simulink library "DAQ_lib_HallPositionTorque"  (R2014b)
settings: Solver=ode45  StartTime=0.0  StopTime=10.0  RelTol=1e-3
undefined symbols (not defined in the file): A_lpf_velocity, ANOMALY_INIT, B1_lpf_velocity, B2_lpf_velocity, Calibration, EnableFT, EncoderAngleLimits, EncoderFiltSys, EncoderThreshold, FTCalibration, GearOffsets, IMUAngleLimits, IMUCommand, IMUThreshold, IMUTorsoOffsets, m_XR17D15x, MAX_ANOMALY, MedullaCommand, MicrostrainFiltSys, MODBUS_TIMEOUT, ResetDAQ, ResetYaw, sample_time, standard, STREAMING_TIMEOUT, TareFT, TorsoCOMOffsets, Ts, TsCAN, TsKVH, UseMicrostrainRate
libraries: xpcethercatlib x207, simulink x53, canmsglib x21, speedgoatlib x13, slrtlib x5, speedgoatlib_IO601 x5, dspswit3 x2, dspmtrx3 x2, xpcseriallib x1, SpeedgoatModified x1
(part 2 of 7)

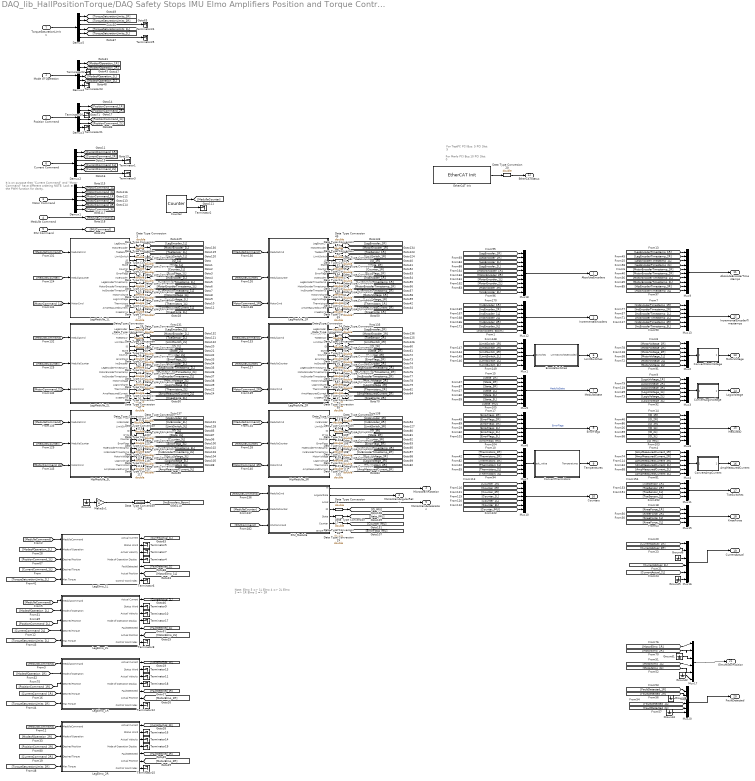
== system DAQ_lib_HallPositionTorque/DAQ Safety Stops IMU Elmo Amplifiers Position and Torque Control with Hall Sensors/DAQ/EtherCATNetwork/EtherCATRobotMicrostrain ==
  note: It is on purpose that "Current Command"
      | and "Motor Command" have different ordering
      | NOTE: Look at the PWM function for clarity.
  note: Note:
      | Elmo 5 => 1L
      | Elmo 4 => 2L
      | Elmo 3 => 1R
      | Elmo 2 => 2R
  note: For Marlo
      | PCI Bus:10 PCI Slot: 0
  note: For TestPC
      | PCI Bus: 5 PCI Slot: 5
  Mode of Operation : Inport
  Position Command : Inport  Port=2
  Motor Command : Inport  Port=3
  Medulla Command : Inport  Port=4
  IMU Command : Inport  Port=5
  Current Command : Inport  Port=6
  TorqueSaturationLimits : Inport  Port=7
  ConvertAmpCurrent : MATLAB Function  TreatAsAtomicUnit=on
  ConvertLogicVoltage : MATLAB Function  TreatAsAtomicUnit=on
  ConvertMotorVoltage : MATLAB Function  TreatAsAtomicUnit=on
  ConvertThermistors : MATLAB Function  TreatAsAtomicUnit=on
  Counter : dspswit3/Counter  Direction=Up  CountEvent=Free running  CounterSize=User defined  MaxCount=65535  InitialCount=0  Output=Count and Hit  HitValue=32  ResetInput=off  SamplesPerFrame=1  Ts=Ts  CntDtype=double  HitDtype=Logical
  Data Type Conversion{1..21,23,25..39,45,47,49..63,69,71,73..87,93,95,98,101..112,114,116..126,141,157} (100 alike) : DataTypeConversion  OutDataTypeStr=double
  Demux{1..5} (5 alike) : Demux  Outputs=6
  EncodeSwitches : MATLAB Function  TreatAsAtomicUnit=on
  "EtherCAT Init " : xpcethercatlib/EtherCAT Init   Priority=0  config_file=C:\Users\rosshart\Desktop\ATRIAS_SVN\MARLO_3D_Controllers\DAQ_withElmos\500us\AllMedullasWithAllMotors_07_08_2015_withBoom.eni.xml  device_id=0  pci_bus=10  pci_slot=0  enaDebug=off  enaDC=on  errLink=off  masterDbg=off  stateChgDbg=off  baseClock=off  masterCfg=off  logFile='c:\dbglog.txt'  sample_time=0.000500
  Ground{,1..6} (7 alike) : Ground
  HipMedulla_3L : Subsystem
  HipMedulla_3R : Subsystem
  IMU_Medulla : Subsystem
  LegElmo_1L : Subsystem
  LegElmo_1R : Subsystem
  LegElmo_2L : Subsystem
  LegElmo_2R : Subsystem
  LegMedulla_1L : Subsystem
  LegMedulla_1R : Subsystem
  LegMedulla_2L : Subsystem
  LegMedulla_2R : Subsystem
  Make3x1 : Gain  Gain=[0; 0; 0]
  Mux{1..4,7,13,16..17,20} (9 alike) : Mux  Inputs=6
  Mux{5..6,8,10,12} (5 alike) : Mux  Inputs=7
  Mux11 : Mux
  Mux15 : Mux
  Mux18 : Mux  Inputs=10
  Mux9 : Mux  Inputs=10
  Terminator{1..25} (25 alike) : Terminator
  AbsoluteEncoders : Outport
  IncrementalEncoders : Outport  Port=2
  MicrostrainRotation : Outport  Port=3
  MicrostrainAngularRate : Outport  Port=4
  MicrostrainAcceleration : Outport  Port=5
  LimitSwitches : Outport  Port=6
  MedullaState : Outport  Port=7
  ErrorFlags : Outport  Port=8
  Temperatures : Outport  Port=9
  Counters : Outport  Port=10
  AbsoluteEncoderTimestamps : Outport  Port=11
  IncrementalEncoderTimestamps : Outport  Port=12
  MotorVoltage : Outport  Port=13
  LogicVoltage : Outport  Port=14
  MedullaID : Outport  Port=15
  AmpMeasuredCurrent : Outport  Port=16
  ToeSwitches : Outport  Port=17
  KneeForce : Outport  Port=18
  CurrentActual : Outport  Port=19
  FaultDetected : Outport  Port=20
  ElmoMotorPosition : Outport  Port=21
  EtherCATStatus : Outport  Port=22
  wires:
  Ground6/1 -> Mux16/3
  Ground5/1 -> Mux16/6
  [CurrentActual_1L] -> Mux16/4
  [CurrentActual_2L] -> Mux16/5
  Ground4/1 -> Mux20/6
  Ground3/1 -> Mux20/3
  [FaultDetected_2L] -> Mux20/5
  [FaultDetected_1L] -> Mux20/4
  Demux4/6 -> Terminator23/1
  Demux4/5 -> [ModeofOperation_2L]
  Demux4/4 -> [ModeofOperation_1L]
  Demux4/3 -> Terminator22/1
  Demux4/1 -> [ModeofOperation_1R]
  Demux4/2 -> [ModeofOperation_2R]
  Demux3/6 -> Terminator21/1
  Demux3/4 -> [PositionCommand_1L]
  Demux3/5 -> [PositionCommand_2L]
  Demux3/3 -> Terminator20/1
  Demux3/1 -> [PositionCommand_1R]
  Demux3/2 -> [PositionCommand_2R]
  Ground2/1 -> Mux17/6
  Ground1/1 -> Mux17/3
  [MotorElmo_1L] -> Mux17/4
  [MotorElmo_2L] -> Mux17/5
  [MotorElmo_2R] -> Mux17/2
  [MotorElmo_1R] -> Mux17/1
  Mux9/1 -> AbsoluteEncoderTimestamps/1
  [HipEncoderTimestamp_3L] -> Mux9/10
  [HipEncoderTimestamp_3R] -> Mux9/9
  [MotorEncoderTimestamp_2L] -> Mux9/8
  [MotorEncoderTimestamp_1L] -> Mux9/7
  [MotorEncoderTimestamp_2R] -> Mux9/6
  [MotorEncoderTimestamp_1R] -> Mux9/5
  [LegEncoderTimestamp_2L] -> Mux9/4
  [LegEncoderTimestamp_1L] -> Mux9/3
  [LegEncoderTimestamp_2R] -> Mux9/2
  [LegEncoderTimestamp_1R] -> Mux9/1
  Mux18/1 -> AbsoluteEncoders/1
  [HipEncoder_3L] -> Mux18/10
  [HipEncoder_3R] -> Mux18/9
  [MotorEncoder_2L] -> Mux18/8
  [MotorEncoder_1L] -> Mux18/7
  [MotorEncoder_2R] -> Mux18/6
  [MotorEncoder_1R] -> Mux18/5
  [LegEncoder_2L] -> Mux18/4
  [LegEncoder_1L] -> Mux18/3
  [LegEncoder_2R] -> Mux18/2
  [LegEncoder_1R] -> Mux18/1
  Mux17/1 -> ElmoMotorPosition/1
  Mux16/1 -> CurrentActual/1
  Current Command/1 -> Demux2/1
  [TorqueSaturationLimits_2R] -> LegElmo_2R/5(Max Torque)
  [TorqueSaturationLimits_1R] -> LegElmo_1R/5(Max Torque)
  [TorqueSaturationLimits_2L] -> LegElmo_2L/5(Max Torque)
  [TorqueSaturationLimits_1L] -> LegElmo_1L/5(Max Torque)
  Mux11/1 -> ToeSwitches/1
  EncodeSwitches/1(LimitSwitchesEncoded) -> LimitSwitches/1
  LegMedulla_1L/2(MotorEncoder) -> Data Type Conversion1/1
  LegMedulla_1L/3(ToeSensor) -> Data Type Conversion2/1
  LegMedulla_1L/4(LimitSwitch) -> Data Type Conversion4/1
  LegMedulla_1L/5(ID) -> Data Type Conversion5/1
  LegMedulla_1L/6(State) -> Data Type Conversion6/1
  LegMedulla_1L/7(Counter) -> Data Type Conversion7/1
  LegMedulla_1L/8(ErrorFlags) -> Data Type Conversion8/1
  LegMedulla_1L/9(IncEncoder) -> Data Type Conversion9/1
  LegMedulla_1L/10(LegEncoderTimestamp) -> Data Type Conversion10/1
  LegMedulla_1L/11(MotorEncoderTimestamp) -> Data Type Conversion11/1
  LegMedulla_1L/12(IncEncoderTimestamp) -> Data Type Conversion12/1
  LegMedulla_1L/13(MotorVoltage) -> Data Type Conversion13/1
  LegMedulla_1L/14(LogicVoltage) -> Data Type Conversion14/1
  LegMedulla_1L/15(Thermistors) -> Data Type Conversion15/1
  LegMedulla_1L/16(AmpMeasuredCurrent) -> Data Type Conversion21/1
  LegMedulla_1L/17(KneeForce) -> Data Type Conversion23/1
  LegMedulla_2L/1(LegEncoder) -> Data Type Conversion25/1
  LegMedulla_2L/2(MotorEncoder) -> Data Type Conversion26/1
  LegMedulla_2L/3(ToeSensor) -> Data Type Conversion27/1
  LegMedulla_2L/4(LimitSwitch) -> Data Type Conversion28/1
  LegMedulla_2L/5(ID) -> Data Type Conversion29/1
  LegMedulla_2L/6(State) -> Data Type Conversion30/1
  LegMedulla_2L/7(Counter) -> Data Type Conversion31/1
  LegMedulla_2L/8(ErrorFlags) -> Data Type Conversion32/1
  LegMedulla_2L/9(IncEncoder) -> Data Type Conversion33/1
  LegMedulla_2L/10(LegEncoderTimestamp) -> Data Type Conversion34/1
  LegMedulla_2L/11(MotorEncoderTimestamp) -> Data Type Conversion35/1
  LegMedulla_2L/12(IncEncoderTimestamp) -> Data Type Conversion36/1
  LegMedulla_2L/13(MotorVoltage) -> Data Type Conversion37/1
  LegMedulla_2L/14(LogicVoltage) -> Data Type Conversion38/1
  LegMedulla_2L/15(Thermistors) -> Data Type Conversion39/1
  LegMedulla_2L/16(AmpMeasuredCurrent) -> Data Type Conversion45/1
  LegMedulla_2L/17(KneeForce) -> Data Type Conversion47/1
  LegMedulla_1R/3(ToeSensor) -> Data Type Conversion51/1
  LegMedulla_1R/4(LimitSwitch) -> Data Type Conversion52/1
  LegMedulla_1R/5(ID) -> Data Type Conversion53/1
  LegMedulla_1R/6(State) -> Data Type Conversion54/1
  LegMedulla_1R/7(Counter) -> Data Type Conversion55/1
  LegMedulla_1R/8(ErrorFlags) -> Data Type Conversion56/1
  LegMedulla_1R/9(IncEncoder) -> Data Type Conversion57/1
  LegMedulla_1R/10(LegEncoderTimestamp) -> Data Type Conversion58/1
  LegMedulla_1R/11(MotorEncoderTimestamp) -> Data Type Conversion59/1
  LegMedulla_1R/12(IncEncoderTimestamp) -> Data Type Conversion60/1
  LegMedulla_1R/13(MotorVoltage) -> Data Type Conversion61/1
  LegMedulla_1R/14(LogicVoltage) -> Data Type Conversion62/1
  LegMedulla_1R/15(Thermistors) -> Data Type Conversion63/1
  LegMedulla_1R/16(AmpMeasuredCurrent) -> Data Type Conversion69/1
  LegMedulla_1R/17(KneeForce) -> Data Type Conversion71/1
  LegMedulla_2R/4(LimitSwitch) -> Data Type Conversion76/1
  LegMedulla_2R/5(ID) -> Data Type Conversion77/1
  LegMedulla_2R/6(State) -> Data Type Conversion78/1
  LegMedulla_2R/7(Counter) -> Data Type Conversion79/1
  LegMedulla_2R/8(ErrorFlags) -> Data Type Conversion80/1
  LegMedulla_2R/9(IncEncoder) -> Data Type Conversion81/1
  LegMedulla_2R/10(LegEncoderTimestamp) -> Data Type Conversion82/1
  LegMedulla_2R/11(MotorEncoderTimestamp) -> Data Type Conversion83/1
  LegMedulla_2R/12(IncEncoderTimestamp) -> Data Type Conversion84/1
  LegMedulla_2R/13(MotorVoltage) -> Data Type Conversion85/1
  LegMedulla_2R/14(LogicVoltage) -> Data Type Conversion86/1
  LegMedulla_2R/15(Thermistor0) -> Data Type Conversion87/1
  LegMedulla_2R/16(AmpMeasuredCurrent) -> Data Type Conversion93/1
  LegMedulla_2R/17(KneeForce) -> Data Type Conversion95/1
  Medulla Command/1 -> [MedullaCommand]
  Counter/2 -> Terminator2/1
  LegMedulla_2R/1(LegEncoder) -> Data Type Conversion73/1
  LegMedulla_2R/2(MotorEncoder) -> Data Type Conversion74/1
  LegMedulla_2R/3(ToeSensor) -> Data Type Conversion75/1
  Data Type Conversion53/1 -> [ID_1R]
  Data Type Conversion54/1 -> [State_1R]
  Data Type Conversion55/1 -> [Counter_1R]
  Data Type Conversion56/1 -> [ErrorFlags_1R]
  Data Type Conversion57/1 -> [IncEncoder_1R]
  Data Type Conversion58/1 -> [LegEncoderTimestamp_1R]
  Data Type Conversion59/1 -> [MotorEncoderTimestamp_1R]
  Data Type Conversion60/1 -> [IncEncoderTimestamp_1R]
  Data Type Conversion61/1 -> [MotorVoltage_1R]
  Data Type Conversion62/1 -> [LogicVoltage_1R]
  Data Type Conversion63/1 -> [Thermistors_1R]
  Data Type Conversion69/1 -> [AmpMeasuredCurrent_1R]
  Data Type Conversion71/1 -> [KneeForce_1R]
  Data Type Conversion77/1 -> [ID_2R]
  Data Type Conversion78/1 -> [State_2R]
  Data Type Conversion79/1 -> [Counter_2R]
  Data Type Conversion80/1 -> [ErrorFlags_2R]
  Data Type Conversion81/1 -> [IncEncoder_2R]
  Data Type Conversion82/1 -> [LegEncoderTimestamp_2R]
  Data Type Conversion83/1 -> [MotorEncoderTimestamp_2R]
  Data Type Conversion84/1 -> [IncEncoderTimestamp_2R]
  Data Type Conversion85/1 -> [MotorVoltage_2R]
  Data Type Conversion86/1 -> [LogicVoltage_2R]
  Data Type Conversion87/1 -> [Thermistors_2R]
  Data Type Conversion93/1 -> [AmpMeasuredCurrent_2R]
  Data Type Conversion95/1 -> [KneeForce_2R]
  Data Type Conversion111/1 -> [AmpMeasuredCurrent_3R]
  LegMedulla_1R/2(MotorEncoder) -> Data Type Conversion50/1
  LegMedulla_1L/1(LegEncoder) -> Data Type Conversion3/1
  LegMedulla_1R/1(LegEncoder) -> Data Type Conversion49/1
  Data Type Conversion5/1 -> [ID_1L]
  Data Type Conversion6/1 -> [State_1L]
  Data Type Conversion7/1 -> [Counter_1L]
  Data Type Conversion29/1 -> [ID_2L]
  Data Type Conversion30/1 -> [State_2L]
  Data Type Conversion31/1 -> [Counter_2L]
  Data Type Conversion32/1 -> [ErrorFlags_2L]
  Data Type Conversion33/1 -> [IncEncoder_2L]
  Data Type Conversion34/1 -> [LegEncoderTimestamp_2L]
  Data Type Conversion35/1 -> [MotorEncoderTimestamp_2L]
  Data Type Conversion36/1 -> [IncEncoderTimestamp_2L]
  Data Type Conversion37/1 -> [MotorVoltage_2L]
  Data Type Conversion38/1 -> [LogicVoltage_2L]
  Data Type Conversion39/1 -> [Thermistors_2L]
  Data Type Conversion45/1 -> [AmpMeasuredCurrent_2L]
  Data Type Conversion47/1 -> [KneeForce_2L]
  Data Type Conversion102/1 -> [Thermistors_3R]
  Data Type Conversion103/1 -> [LogicVoltage_3R]
  Data Type Conversion101/1 -> [MotorVoltage_3R]
  Data Type Conversion108/1 -> [IncEncoderTimestamp_3R]
  Data Type Conversion109/1 -> [HipEncoderTimestamp_3R]
  Data Type Conversion104/1 -> [IncEncoder_3R]
  Data Type Conversion106/1 -> [ErrorFlags_3R]
  Data Type Conversion107/1 -> [Counter_3R]
  Data Type Conversion105/1 -> [State_3R]
  Data Type Conversion110/1 -> [ID_3R]
  Data Type Conversion98/1 -> [HipEncoder_3R]
  HipMedulla_3R/1(HipEncoder) -> Data Type Conversion98/1
  HipMedulla_3R/2(IncEncoder) -> Data Type Conversion104/1
  HipMedulla_3R/3(LimitSwitch) -> Data Type Conversion157/1
  HipMedulla_3R/4(ID) -> Data Type Conversion110/1
  HipMedulla_3R/5(State) -> Data Type Conversion105/1
  HipMedulla_3R/6(Counter) -> Data Type Conversion107/1
  HipMedulla_3R/7(ErrorFlags) -> Data Type Conversion106/1
  HipMedulla_3R/8(HipEncoderTimestamp) -> Data Type Conversion109/1
  HipMedulla_3R/9(IncEncoderTimestamp) -> Data Type Conversion108/1
  HipMedulla_3R/10(MotorVoltage) -> Data Type Conversion101/1
  HipMedulla_3R/11(LogicVoltage) -> Data Type Conversion103/1
  HipMedulla_3R/12(Thermistors) -> Data Type Conversion102/1
  HipMedulla_3R/13(AmpMeasuredCurrent) -> Data Type Conversion111/1
  HipMedulla_3L/3(LimitSwitch) -> Data Type Conversion112/1
  Data Type Conversion114/1 -> [HipEncoder_3L]
  HipMedulla_3L/1(HipEncoder) -> Data Type Conversion114/1
  HipMedulla_3L/2(IncEncoder) -> Data Type Conversion119/1
  Data Type Conversion126/1 -> [AmpMeasuredCurrent_3L]
  Data Type Conversion117/1 -> [Thermistors_3L]
  Data Type Conversion118/1 -> [LogicVoltage_3L]
  Data Type Conversion116/1 -> [MotorVoltage_3L]
  Data Type Conversion123/1 -> [IncEncoderTimestamp_3L]
  Data Type Conversion124/1 -> [HipEncoderTimestamp_3L]
  Data Type Conversion119/1 -> [IncEncoder_3L]
  Data Type Conversion121/1 -> [ErrorFlags_3L]
  Data Type Conversion122/1 -> [Counter_3L]
  Data Type Conversion120/1 -> [State_3L]
  Data Type Conversion125/1 -> [ID_3L]
  HipMedulla_3L/4(ID) -> Data Type Conversion125/1
  HipMedulla_3L/5(State) -> Data Type Conversion120/1
  HipMedulla_3L/6(Counter) -> Data Type Conversion122/1
  HipMedulla_3L/7(ErrorFlags) -> Data Type Conversion121/1
  HipMedulla_3L/8(HipEncoderTimestamp) -> Data Type Conversion124/1
  HipMedulla_3L/9(IncEncoderTimestamp) -> Data Type Conversion123/1
  HipMedulla_3L/10(MotorVoltage) -> Data Type Conversion116/1
  HipMedulla_3L/11(LogicVoltage) -> Data Type Conversion118/1
  HipMedulla_3L/12(Thermistors) -> Data Type Conversion117/1
  HipMedulla_3L/13(AmpMeasuredCurrent) -> Data Type Conversion126/1
  Mux1/1 -> EncodeSwitches/1(Switches)
  Data Type Conversion8/1 -> [ErrorFlags_1L]
  Data Type Conversion9/1 -> [IncEncoder_1L]
  Data Type Conversion10/1 -> [LegEncoderTimestamp_1L]
  Data Type Conversion11/1 -> [MotorEncoderTimestamp_1L]
  Data Type Conversion12/1 -> [IncEncoderTimestamp_1L]
  Data Type Conversion13/1 -> [MotorVoltage_1L]
  Data Type Conversion14/1 -> [LogicVoltage_1L]
  Data Type Conversion15/1 -> [Thermistors_1L]
  Data Type Conversion21/1 -> [AmpMeasuredCurrent_1L]
  Data Type Conversion23/1 -> [KneeForce_1L]
  [MotorVoltage_1R] -> Mux2/1
  [MotorVoltage_2R] -> Mux2/2
  [MotorVoltage_3R] -> Mux2/3
  [MotorVoltage_1L] -> Mux2/4
  [MotorVoltage_2L] -> Mux2/5
  [MotorVoltage_3L] -> Mux2/6
  [LogicVoltage_1R] -> Mux3/1
  [LogicVoltage_2R] -> Mux3/2
  [LogicVoltage_3R] -> Mux3/3
  [LogicVoltage_1L] -> Mux3/4
  [LogicVoltage_2L] -> Mux3/5
  [LogicVoltage_3L] -> Mux3/6
  [AmpMeasuredCurrent_1R] -> Mux4/1
  [AmpMeasuredCurrent_2R] -> Mux4/2
  [AmpMeasuredCurrent_3R] -> Mux4/3
  [AmpMeasuredCurrent_1L] -> Mux4/4
  [AmpMeasuredCurrent_2L] -> Mux4/5
  [AmpMeasuredCurrent_3L] -> Mux4/6
  [State_1R] -> Mux5/1
  [State_2R] -> Mux5/2
  [State_3R] -> Mux5/3
  [State_1L] -> Mux5/4
  [State_2L] -> Mux5/5
  [State_3L] -> Mux5/6
  [ErrorFlags_1R] -> Mux6/1
  [ErrorFlags_2R] -> Mux6/2
  [ErrorFlags_3R] -> Mux6/3
  [ErrorFlags_1L] -> Mux6/4
  [ErrorFlags_2L] -> Mux6/5
  [ErrorFlags_3L] -> Mux6/6
  [ErrorFlags_IMU] -> Mux6/7
  [State_IMU] -> Mux5/7
  Mux2/1 -> ConvertMotorVoltage/1(adc_value)
  Mux3/1 -> ConvertLogicVoltage/1(adc_value)
  Mux4/1 -> ConvertAmpCurrent/1(adc_value)
  ConvertMotorVoltage/1(motorVoltage) -> MotorVoltage/1
  ConvertLogicVoltage/1(logicVoltage) -> LogicVoltage/1
  ConvertAmpCurrent/1(measuredCurrent) -> AmpMeasuredCurrent/1
  Mux5/1 -> MedullaState/1  "MedullaState"
  Mux6/1 -> ErrorFlags/1  "ErrorFlags"
  Mux10/1 -> Counters/1
  [Counter_1R] -> Mux10/1
  [Counter_2R] -> Mux10/2
  [Counter_3R] -> Mux10/3
  [Counter_1L] -> Mux10/4
  [Counter_2L] -> Mux10/5
  [Counter_3L] -> Mux10/6
  [Counter_IMU] -> Mux10/7
  Counter/1 -> [MedullaCounter]
  [MedullaCounter] -> LegMedulla_1L/2(MedullaCounter)
  [MedullaCounter] -> HipMedulla_3L/2(MedullaCounter)
  [MedullaCounter] -> HipMedulla_3R/2(MedullaCounter)
  [MedullaCounter] -> LegMedulla_2R/2(MedullaCounter)
  [MedullaCounter] -> LegMedulla_1R/2(MedullaCounter)
  [MedullaCounter] -> LegMedulla_2L/2(MedullaCounter)
  [MedullaCommand] -> LegMedulla_1R/1(MedullaCmd)
  [MedullaCommand] -> LegMedulla_2R/1(MedullaCmd)
  [MedullaCommand] -> LegMedulla_2L/1(MedullaCmd)
  [MedullaCommand] -> LegMedulla_1L/1(MedullaCmd)
  [MedullaCommand] -> HipMedulla_3R/1(MedullaCmd)
  [MedullaCommand] -> HipMedulla_3L/1(MedullaCmd)
  [MotorCommand_1L] -> LegMedulla_1L/3(MotorCmd)
  [MotorCommand_2L] -> LegMedulla_2L/3(MotorCmd)
  [MotorCommand_1R] -> LegMedulla_1R/3(MotorCmd)
  [MotorCommand_2R] -> LegMedulla_2R/3(MotorCmd)
  [MotorCommand_3R] -> HipMedulla_3R/3(MotorCmd)
  Demux1/6 -> [MotorCommand_3L]
  [MotorCommand_3L] -> HipMedulla_3L/3(MotorCmd)
  Demux1/1 -> [MotorCommand_1L]
  Demux1/2 -> [MotorCommand_2L]
  Demux1/3 -> [MotorCommand_1R]
  Demux1/4 -> [MotorCommand_2R]
  Demux1/5 -> [MotorCommand_3R]
  Data Type Conversion157/1 -> [LimitSwitch_3R]
  Data Type Conversion112/1 -> [LimitSwitch_3L]
  [LimitSwitch_1R] -> Mux1/1
  [LimitSwitch_2R] -> Mux1/2
  [LimitSwitch_3R] -> Mux1/3
  [LimitSwitch_1L] -> Mux1/4
  [LimitSwitch_2L] -> Mux1/5
  [LimitSwitch_3L] -> Mux1/6
  [ToeSensor_1R] -> Mux11/1
  [ToeSensor_2R] -> Mux11/2
  [ToeSensor_1L] -> Mux11/3
  [ToeSensor_2L] -> Mux11/4
  Data Type Conversion76/1 -> [LimitSwitch_2R]
  Data Type Conversion75/1 -> [ToeSensor_2R]
  Data Type Conversion51/1 -> [ToeSensor_1R]
  Data Type Conversion52/1 -> [LimitSwitch_1R]
  Data Type Conversion27/1 -> [ToeSensor_2L]
  Data Type Conversion28/1 -> [LimitSwitch_2L]
  Data Type Conversion2/1 -> [ToeSensor_1L]
  Data Type Conversion4/1 -> [LimitSwitch_1L]
  Data Type Conversion3/1 -> [LegEncoder_1L]
  Data Type Conversion1/1 -> [MotorEncoder_1L]
  Data Type Conversion25/1 -> [LegEncoder_2L]
  Data Type Conversion26/1 -> [MotorEncoder_2L]
  Data Type Conversion49/1 -> [LegEncoder_1R]
  Data Type Conversion50/1 -> [MotorEncoder_1R]
  Data Type Conversion73/1 -> [LegEncoder_2R]
  Data Type Conversion74/1 -> [MotorEncoder_2R]
  [IncEncoder_1R] -> Mux12/1
  [IncEncoder_2R] -> Mux12/2
  [IncEncoder_3R] -> Mux12/5
  [IncEncoder_1L] -> Mux12/3
  [IncEncoder_2L] -> Mux12/4
  [IncEncoder_3L] -> Mux12/6
  IMU Command/1 -> [IMUCommand]
  [MedullaCommand] -> IMU_Medulla/1(MedullaCmd)
  [MedullaCounter] -> IMU_Medulla/2(MedullaCounter)
  [IMUCommand] -> IMU_Medulla/3(IMUCommand)
  IMU_Medulla/1(M) -> MicrostrainRotation/1
  IMU_Medulla/4(ID) -> Data Type Conversion16/1
  IMU_Medulla/5(State) -> Data Type Conversion17/1
  IMU_Medulla/6(Counter) -> Data Type Conversion18/1
  IMU_Medulla/7(ErrorFlags) -> Data Type Conversion19/1
  Mux7/1 -> ConvertThermistors/1(adc_value)
  ConvertThermistors/1(Temperatures) -> Temperatures/1
  Motor Command/1 -> Demux1/1
  [Thermistors_1R] -> Mux7/1
  [Thermistors_2L] -> Mux7/5
  [Thermistors_1L] -> Mux7/4
  [Thermistors_2R] -> Mux7/2
  [Thermistors_3L] -> Mux7/6
  [Thermistors_3R] -> Mux7/3
  Mux12/1 -> IncrementalEncoders/1
  [ID_2L] -> Mux8/5
  [ID_IMU] -> Mux8/7
  [ID_1L] -> Mux8/4
  [ID_1R] -> Mux8/1
  [ID_2R] -> Mux8/2
  [ID_3R] -> Mux8/3
  [ID_3L] -> Mux8/6
  Mux8/1 -> MedullaID/1
  Data Type Conversion141/1 -> [IncEncoders_Boom]
  Mux13/1 -> IncrementalEncoderTimestamps/1
  [IncEncoderTimestamp_3R] -> Mux13/5
  [IncEncoderTimestamp_1R] -> Mux13/1
  [IncEncoderTimestamp_1L] -> Mux13/3
  [IncEncoderTimestamp_2L] -> Mux13/4
  [IncEncoderTimestamp_2R] -> Mux13/2
  [IncEncoderTimestamp_3L] -> Mux13/6
  Mux15/1 -> KneeForce/1
  [KneeForce_1R] -> Mux15/1
  [KneeForce_2R] -> Mux15/2
  [KneeForce_1L] -> Mux15/3
  [KneeForce_2L] -> Mux15/4
  IMU_Medulla/3(Accel) -> MicrostrainAcceleration/1
  IMU_Medulla/2(AngularRate) -> MicrostrainAngularRate/1
  Ground/1 -> Make3x1/1
  Make3x1/1 -> Data Type Conversion141/1
  [IncEncoders_Boom] -> Mux12/7
  Data Type Conversion16/1 -> [ID_IMU]
  Data Type Conversion17/1 -> [State_IMU]
  Data Type Conversion18/1 -> [Counter_IMU]
  Data Type Conversion19/1 -> [ErrorFlags_IMU]
  [MedullaCommand] -> LegElmo_1L/1(MedullaCommand)
  [CurrentActual_1R] -> Mux16/1
  [CurrentActual_2R] -> Mux16/2
  Mux20/1 -> FaultDetected/1
  [FaultDetected_1R] -> Mux20/1
  [FaultDetected_2R] -> Mux20/2
  LegElmo_1L/3(Actual Velocity) -> Terminator7/1
  LegElmo_1L/5(FaultDetected) -> [FaultDetected_1L]
  Demux2/1 -> [CurrentCommand_1R]
  Demux2/5 -> [CurrentCommand_2L]
  Demux2/2 -> [CurrentCommand_2R]
  Demux2/3 -> Terminator1/1
  Demux2/4 -> [CurrentCommand_1L]
  Demux2/6 -> Terminator3/1
  Position Command/1 -> Demux3/1
  LegElmo_1L/4(Mode of Operation Display) -> Terminator4/1
  LegElmo_1L/2(Status Word) -> Terminator5/1
  LegElmo_1L/7(Control Word Index) -> Terminator6/1
  LegElmo_1L/1(Actual Current) -> [CurrentActual_1L]
  [CurrentCommand_1L] -> LegElmo_1L/4(Desired Torque)
  [MedullaCommand] -> LegElmo_2L/1(MedullaCommand)
  [MedullaCommand] -> LegElmo_1R/1(MedullaCommand)
  [MedullaCommand] -> LegElmo_2R/1(MedullaCommand)
  [CurrentCommand_2R] -> LegElmo_2R/4(Desired Torque)
  LegElmo_2L/2(Status Word) -> Terminator9/1
  LegElmo_2L/3(Actual Velocity) -> Terminator10/1
  [CurrentCommand_2L] -> LegElmo_2L/4(Desired Torque)
  LegElmo_1R/2(Status Word) -> Terminator13/1
  LegElmo_1R/3(Actual Velocity) -> Terminator11/1
  LegElmo_2R/2(Status Word) -> Terminator16/1
  LegElmo_2R/3(Actual Velocity) -> Terminator14/1
  LegElmo_2L/1(Actual Current) -> [CurrentActual_2L]
  LegElmo_2R/1(Actual Current) -> [CurrentActual_2R]
  LegElmo_1R/1(Actual Current) -> [CurrentActual_1R]
  LegElmo_2L/7(Control Word Index) -> Terminator8/1
  LegElmo_1R/7(Control Word Index) -> Terminator12/1
  LegElmo_2R/7(Control Word Index) -> Terminator15/1
  LegElmo_2L/4(Mode of Operation Display) -> Terminator17/1
  LegElmo_1R/4(Mode of Operation Display) -> Terminator18/1
  LegElmo_2R/4(Mode of Operation Display) -> Terminator19/1
  LegElmo_2L/5(FaultDetected) -> [FaultDetected_2L]
  LegElmo_1R/5(FaultDetected) -> [FaultDetected_1R]
  LegElmo_2R/5(FaultDetected) -> [FaultDetected_2R]
  [PositionCommand_1L] -> LegElmo_1L/3(Desired Position)
  [PositionCommand_2L] -> LegElmo_2L/3(Desired Position)
  [PositionCommand_1R] -> LegElmo_1R/3(Desired Position)
  [PositionCommand_2R] -> LegElmo_2R/3(Desired Position)
  LegElmo_1L/6(Actual Position) -> [MotorElmo_1L]
  LegElmo_2L/6(Actual Position) -> [MotorElmo_2L]
  LegElmo_1R/6(Actual Position) -> [MotorElmo_1R]
  LegElmo_2R/6(Actual Position) -> [MotorElmo_2R]
  Mode of Operation/1 -> Demux4/1
  [ModeofOperation_1L] -> LegElmo_1L/2(Mode of Operation)
  [ModeofOperation_2L] -> LegElmo_2L/2(Mode of Operation)
  [ModeofOperation_1R] -> LegElmo_1R/2(Mode of Operation)
  [ModeofOperation_2R] -> LegElmo_2R/2(Mode of Operation)
  TorqueSaturationLimits/1 -> Demux5/1
  Demux5/1 -> [TorqueSaturationLimits_1R]
  Demux5/5 -> [TorqueSaturationLimits_2L]
  Demux5/2 -> [TorqueSaturationLimits_2R]
  Demux5/3 -> Terminator24/1
  Demux5/4 -> [TorqueSaturationLimits_1L]
  Demux5/6 -> Terminator25/1
  [CurrentCommand_1R] -> LegElmo_1R/4(Desired Torque)
  Data Type Conversion20/1 -> EtherCATStatus/1
  "EtherCAT Init "/1 -> Data Type Conversion20/1

== system DAQ_lib_HallPositionTorque/DAQ Safety Stops IMU Elmo Amplifiers Position and Torque Control with Hall Sensors/DAQ/EtherCATNetwork/IMUFilters ==
  q : Inport  Partition=on  PartitionDimension=1  PartitionWidth=1
  q_limits : Inport  Port=2  Partition=on  PartitionDimension=1  PartitionWidth=1
  Threshold : Inport  Port=3  Partition=off
  Reset : Inport  Port=4  Partition=off
  IMURate : Inport  Port=5  Partition=on  PartitionDimension=1  PartitionWidth=1
  UseIMURate : Inport  Port=6  Partition=off
  CheckAndFilterIMU : Subsystem
  For Each : ForEach  DisableCoverage=on  IndexMode=One-based
  q_clean : Outport  ConcatenationDimension=1
  dq_clean : Outport  Port=2  ConcatenationDimension=1
  ErrorCount : Outport  Port=3  ConcatenationDimension=1
  wires:
  UseIMURate/1 -> CheckAndFilterIMU/6(UseIMURate)
  IMURate/1 -> CheckAndFilterIMU/5(IMURate)
  q/1 -> CheckAndFilterIMU/1(q_daq)
  Threshold/1 -> CheckAndFilterIMU/3(Threshold)
  CheckAndFilterIMU/1(q_clean) -> q_clean/1
  CheckAndFilterIMU/3(ErrorCount) -> ErrorCount/1
  q_limits/1 -> CheckAndFilterIMU/2(q_limits)
  CheckAndFilterIMU/2(dq_clean) -> dq_clean/1
  Reset/1 -> CheckAndFilterIMU/4(Reset)

== system DAQ_lib_HallPositionTorque/DAQ Safety Stops IMU Elmo Amplifiers Position and Torque Control with Hall Sensors/DAQ/EtherCATNetwork/Subsystem ==
  Temp : Inport
  Counter : dspswit3/Counter  Direction=Up  CountEvent=Free running  CounterSize=User defined  MaxCount=29  InitialCount=0  Output=Count  HitValue=32  ResetInput=off  SamplesPerFrame=1  Ts=0.0005  CntDtype=uint8  HitDtype=Logical
  Discrete Filter : DiscreteFilter  Numerator=[1-0.99]  Denominator=[1 -0.99]  InitialStates=zeros(30,1)
  Index Vector : MultiPortSwitch  DataPortOrder=Zero-based contiguous  Inputs=1  zeroidx=on
  MxTemp : Outport
  wires:
  Temp/1 -> Discrete Filter/1
  Index Vector/1 -> MxTemp/1
  Discrete Filter/1 -> Index Vector/2
  Counter/1 -> Index Vector/1

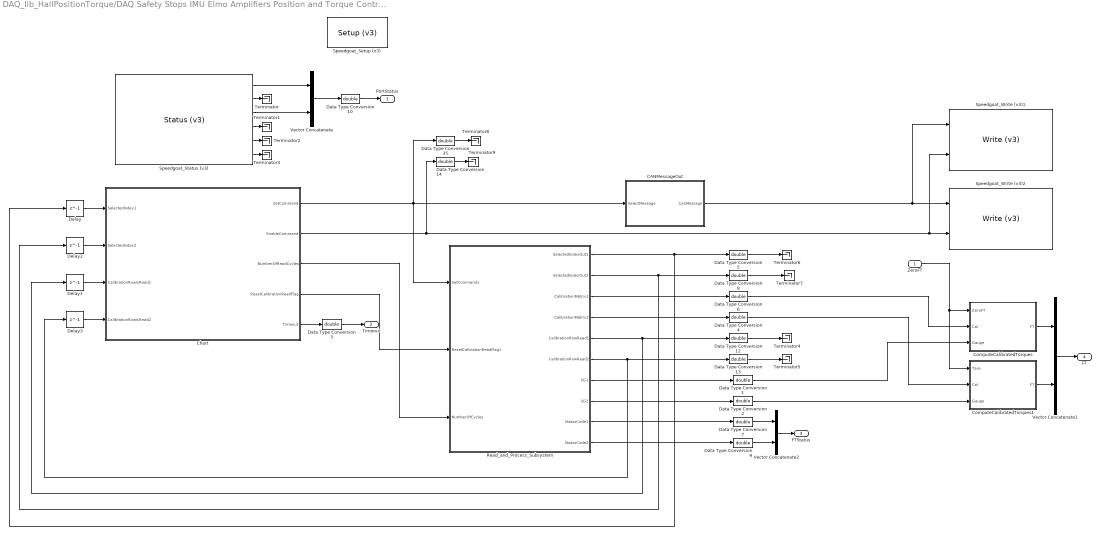
== system DAQ_lib_HallPositionTorque/DAQ Safety Stops IMU Elmo Amplifiers Position and Torque Control with Hall Sensors/DAQ/SerialInterfaces/FTCAN ==
  ZeroFT : Inport
  CANMessageOut : Subsystem
  Chart : Stateflow chart  TreatAsAtomicUnit=on
  ComputeCalibratedTorques : Subsystem
  ComputeCalibratedTorques1 : Subsystem
  Data Type Conversion{1..10,12..14,35} (14 alike) : DataTypeConversion  OutDataTypeStr=double
  Delay{,1..3} (4 alike) : Delay  DelayLength=1  InitialCondition=0
  Read_and_Process_Subsystem : Subsystem
  Speedgoat_Setup (v3) : speedgoatlib_IO601/Setup (v3)  id=1  can1enable=on  can1bus=Highspeed  can1Baudrate=250 kBaud  can1UserBR=[1,1,5,2]  stdAcc1=[0,0,0,0]  extAcc1=[0,0,0,0]  can2enable=on  can2bus=Highspeed  can2Baudrate=250 kBaud  can2UserBR=[1,1,5,2]  stdAcc2=[0,0,0,0]  extAcc2=[0,0,0,0]  pciSlot=-1
  Speedgoat_Status (v3) : speedgoatlib_IO601/Status (v3)  id=1  ts=-1  pciSlot=-1
  Speedgoat_Write (v3)1 : speedgoatlib_IO601/Write (v3)  Priority=1  id=1  sampletime=-1  pciSlot=-1  inputType=CAN_MESSAGE plus count  port=1  maxMsg=1  status=off  init=[]  term=[]
  Speedgoat_Write (v3)2 : speedgoatlib_IO601/Write (v3)  Priority=1  id=1  sampletime=-1  pciSlot=-1  inputType=CAN_MESSAGE plus count  port=2  maxMsg=1  status=off  init=[]  term=[]
  Terminator{,1..9} (10 alike) : Terminator
  Vector Concatenate : Concatenate
  Vector Concatenate1 : Concatenate
  Vector Concatenate2 : Concatenate
  PortStatus : Outport
  Timeout : Outport  Port=2
  FTStatus : Outport  Port=3
  FT : Outport  Port=4
  wires:
  CANMessageOut/1(CanMessage) -> Speedgoat_Write (v3)2/1, Speedgoat_Write (v3)1/1
  Data Type Conversion35/1 -> Terminator8/1
  Chart/2(EnableCommand) -> Data Type Conversion14/1, Speedgoat_Write (v3)1/2, Speedgoat_Write (v3)2/2
  Read_and_Process_Subsystem/3(CalibrationMatrix1) -> Data Type Conversion6/1
  Data Type Conversion6/1 -> ComputeCalibratedTorques/2(Cal)
  Chart/4(ResetCalibrationReadFlag) -> Read_and_Process_Subsystem/2(ResetCalbrationReadFlag1)
  Read_and_Process_Subsystem/1(SelectedIndexOut1) -> Data Type Conversion5/1, Delay/1
  Delay1/1 -> Chart/3(CalibrationRowIsRead1)
  Delay/1 -> Chart/1(SelectedIndex1)
  Data Type Conversion1/1 -> ComputeCalibratedTorques/3(Gauge)
  Data Type Conversion3/1 -> Timeout/1
  Chart/5(Timeout) -> Data Type Conversion3/1
  Delay2/1 -> Chart/2(SelectedIndex2)
  Read_and_Process_Subsystem/2(SelectedIndexOut2) -> Data Type Conversion8/1, Delay2/1
  Data Type Conversion2/1 -> ComputeCalibratedTorques1/3(Gauge)
  Read_and_Process_Subsystem/4(CalibrationMatrix2) -> Data Type Conversion4/1
  Data Type Conversion4/1 -> ComputeCalibratedTorques1/2(Cal)
  Read_and_Process_Subsystem/7(SG1) -> Data Type Conversion1/1
  Read_and_Process_Subsystem/8(SG2) -> Data Type Conversion2/1
  Delay3/1 -> Chart/4(CalibrationRowIsRead2)
  Read_and_Process_Subsystem/6(CalibrationRowRead2) -> Data Type Conversion13/1, Delay3/1
  Data Type Conversion5/1 -> Terminator6/1
  Data Type Conversion8/1 -> Terminator7/1
  Data Type Conversion7/1 -> Vector Concatenate2/1
  Read_and_Process_Subsystem/9(StatusCode1) -> Data Type Conversion7/1
  Data Type Conversion9/1 -> Vector Concatenate2/2
  Read_and_Process_Subsystem/10(StatusCode2) -> Data Type Conversion9/1
  Read_and_Process_Subsystem/5(CalibrationRowRead1) -> Data Type Conversion12/1, Delay1/1
  Data Type Conversion10/1 -> PortStatus/1
  Speedgoat_Status (v3)/1 -> Vector Concatenate/1
  Speedgoat_Status (v3)/3 -> Vector Concatenate/2
  Chart/3(NumberOfReadCycles) -> Read_and_Process_Subsystem/3(NumberOfCycles)
  Chart/1(SetCommand) -> Data Type Conversion35/1, CANMessageOut/1(SelectMessage), Read_and_Process_Subsystem/1(SetCommand1)
  Data Type Conversion14/1 -> Terminator9/1
  Speedgoat_Status (v3)/4 -> Terminator1/1
  Speedgoat_Status (v3)/6 -> Terminator3/1
  Speedgoat_Status (v3)/5 -> Terminator2/1
  Speedgoat_Status (v3)/2 -> Terminator/1
  Vector Concatenate/1 -> Data Type Conversion10/1
  ComputeCalibratedTorques/1(FT) -> Vector Concatenate1/1
  Vector Concatenate1/1 -> FT/1
  ComputeCalibratedTorques1/1(FT) -> Vector Concatenate1/2
  ZeroFT/1 -> ComputeCalibratedTorques/1(ZeroFT), ComputeCalibratedTorques1/1(Tare)
  Vector Concatenate2/1 -> FTStatus/1
  Data Type Conversion12/1 -> Terminator4/1
  Data Type Conversion13/1 -> Terminator5/1

== system DAQ_lib_HallPositionTorque/DAQ Safety Stops IMU Elmo Amplifiers Position and Torque Control with Hall Sensors/DAQ/SerialInterfaces/FTInterface ==
  Tare : Inport
  Reset : Inport  Port=2
  Enable : EnablePort
  ATI Serial NoInt : Subsystem  mask{irqnum=9, slot=[4 5]}
      mask prompts: irqnum "IRQ"; slot "PCI [bus slot]"
      mask TypeOptions irqnum: 5 | 9
      mask Callback irqnum: set_param([gcb '/Board Setup'], 'irqnum', num2str(get_param(gcb,'irqnum')));
      mask Display:
      | disp('IO503\nTPMC466\nSend Interrupt-Free\nReceive Interrup-Free')
      | 
      | port_label('input', 1, 'TX1')
      | port_label('input', 2, 'TX2')
      | 
      | port_label('output', 1, 'RX1')
      | port_label('output', 2, 'RX2')
  CalibrationSet : Constant
  Demux : Demux  Outputs=2
  Mux : Mux  Inputs=2
  Subsystem : Subsystem
  FTStatus : Outport  OutputWhenDisabled=reset  InitialOutput=zeros(2,1)
  FT : Outport  Port=2  OutputWhenDisabled=reset  InitialOutput=zeros(12,1)
  FTInterfaceStatus : Outport  Port=3  OutputWhenDisabled=reset  InitialOutput=zeros(2,1)
  FTSetupStatus : Outport  Port=4  OutputWhenDisabled=reset  InitialOutput=zeros(2,1)
  CalibrationSerial : Outport  Port=5  OutputWhenDisabled=reset  InitialOutput=zeros(2,1)
  wires:
  Subsystem/4(FTSetupStatus) -> FTSetupStatus/1
  Subsystem/3(FTInterfaceStatus) -> FTInterfaceStatus/1
  Subsystem/5(CalibrationSerial) -> CalibrationSerial/1
  CalibrationSet/1 -> Subsystem/1(CalibrationSet)
  Subsystem/2(FT) -> FT/1
  ATI Serial NoInt/2(RX2) -> Mux/2
  Subsystem/1(FTStatus) -> FTStatus/1
  Tare/1 -> Subsystem/2(Tare)
  Reset/1 -> Subsystem/3(Reset)
  Mux/1 -> Subsystem/4(SerialIn)
  Subsystem/6(SerialOut) -> Demux/1
  Demux/2 -> ATI Serial NoInt/2(TX2)
  Demux/1 -> ATI Serial NoInt/1(TX1)
  ATI Serial NoInt/1(RX1) -> Mux/1

== system DAQ_lib_HallPositionTorque/DAQ Safety Stops IMU Elmo Amplifiers Position and Torque Control with Hall Sensors/DAQ/SerialInterfaces/KVH ==
  ResetYaw : Inport
  Reset : Inport  Port=2
  ComputeEulerAngles : MATLAB Function  TreatAsAtomicUnit=on
  KVHOrientation : Constant  Value=Calibration.KVHOrientation
  Logical Operator : Logic  Operator=OR  OutDataTypeStr=boolean
  Reshape : Reshape
  Send Receive1 : Subsystem  Commented=on  InitFcn=m_XR17D15x(3);  mask(sendreceive_IO503){slot=[4 5], irqnum=9}
      mask prompts: slot "PCI slot (-1: autosearch):"; irqnum "IRQ number:"
      mask help:
      | Speedgoat driver block
      | IO503 - Send Receive
      mask Help: web(fullfile(speedgoatroot,'sg_help','serial','dialog_fields_send_rec_io503.htm'),'-helpbrowser');
      mask Display:
      | disp('Speedgoat\nIO503\n422 Receive\nNo Interrupts');
      | 
      | port_label( 'output', 1, 'Rx3' );
  Subsystem : Subsystem  mask{irqnum=5, slot=[4 4]}
      mask prompts: irqnum "IRQ"; slot "PCI [bus slot]"
      mask TypeOptions irqnum: 5 | 9
      mask Callback irqnum: set_param([gcb '/Board Setup'], 'irqnum', num2str(get_param(gcb,'irqnum')));
      mask Display:
      | disp('Speedgoat\nIO503\nRS422 Receive\nInterrupt-free');
      | port_label( 'output', 1, 'RX3' );
  Unit Delay1 : UnitDelay  InitialCondition=[0; 0]  SampleTime=-1
  Unit Delay2 : UnitDelay  InitialCondition=zeros(3,3)  SampleTime=-1
  UpdateOrientation : Subsystem
  EulerAngles : Outport
  EulerAngleDerivatives : Outport  Port=2
  Rk : Outport  Port=3
  DeltaAngle : Outport  Port=4
  Accel : Outport  Port=5
  Status : Outport  Port=6
  Sequence : Outport  Port=7
  Temperature : Outport  Port=8
  Valid : Outport  Port=9
  PacketSize : Outport  Port=10
  wires:
  [Reset] -> UpdateOrientation/2(Reset)
  UpdateOrientation/5(Status) -> Status/1
  UpdateOrientation/7(Temperature) -> Temperature/1
  UpdateOrientation/4(Acceleration) -> Accel/1
  UpdateOrientation/3(DeltaAngle) -> DeltaAngle/1
  UpdateOrientation/8(Valid) -> Valid/1
  UpdateOrientation/6(Sequence) -> Sequence/1
  Reset/1 -> [Reset]
  KVHOrientation/1 -> ComputeEulerAngles/3(RCal)
  Unit Delay2/1 -> ComputeEulerAngles/5(R0In)
  ComputeEulerAngles/1(ZYX) -> EulerAngles/1
  ComputeEulerAngles/4(R0) -> Unit Delay2/1
  ComputeEulerAngles/3(Rk) -> Reshape/1
  [Reset] -> Logical Operator/1
  Reshape/1 -> Rk/1
  UpdateOrientation/1(Rk) -> ComputeEulerAngles/1(RkIn)
  UpdateOrientation/2(wk) -> ComputeEulerAngles/2(wk)
  ComputeEulerAngles/2(dZYX) -> EulerAngleDerivatives/1
  ComputeEulerAngles/5(YawRollover) -> Unit Delay1/1
  Unit Delay1/1 -> ComputeEulerAngles/6(YawRolloverIn)
  ResetYaw/1 -> Logical Operator/2
  Logical Operator/1 -> ComputeEulerAngles/4(Reset)
  Subsystem/1(SerialData) -> UpdateOrientation/1(FIFO)
  UpdateOrientation/9(PacketSize) -> PacketSize/1

== system DAQ_lib_HallPositionTorque/DAQ Safety Stops IMU Elmo Amplifiers Position and Torque Control with Hall Sensors/DAQ/EtherCATNetwork/EncoderFilters/CheckAndFilterEncoder ==
  q_daq : Inport
  q_limits : Inport  Port=2
  Threshold : Inport  Port=3
  Reset : Inport  Port=4
  Counter : Inport  Port=5
  AnomalyDetection : Stateflow chart  TreatAsAtomicUnit=on  SystemSampleTime=EncoderFiltSys.dt
  Constant : Constant  Value=EncoderFiltSys.dt
  Discrete State-Space : DiscreteStateSpace  A=EncoderFiltSys.A  B=EncoderFiltSys.B  C=EncoderFiltSys.C  D=EncoderFiltSys.D  X0=EncoderFiltSys.x0  SampleTime=EncoderFiltSys.dt
  OSU_filter : Subsystem
  Unit Delay : UnitDelay  SampleTime=EncoderFiltSys.dt
  q_clean : Outport
  dq_clean : Outport  Port=2
  ErrorCount : Outport  Port=3
  wires:
  Counter/1 -> AnomalyDetection/3(Counter)
  Reset/1 -> AnomalyDetection/6(Reset)
  AnomalyDetection/2(ErrorCount) -> ErrorCount/1
  q_limits/1 -> AnomalyDetection/4(q_limits)
  Constant/1 -> AnomalyDetection/7(ANOMALY_DT)
  Unit Delay/1 -> AnomalyDetection/2(dq)
  Threshold/1 -> AnomalyDetection/5(Threshold)
  q_daq/1 -> AnomalyDetection/1(q)
  AnomalyDetection/1(q_clean) -> OSU_filter/1(q), q_clean/1, Discrete State-Space/1
  Discrete State-Space/1 -> Unit Delay/1
  OSU_filter/1(dq) -> dq_clean/1

== system DAQ_lib_HallPositionTorque/DAQ Safety Stops IMU Elmo Amplifiers Position and Torque Control with Hall Sensors/DAQ/EtherCATNetwork/EtherCATRobotMicrostrain/HipMedulla_3L ==
  MedullaCmd : Inport
  MedullaCounter : Inport  Port=2
  MotorCmd : Inport  Port=3
  Data Type Conversion3 : DataTypeConversion  OutDataTypeStr=uint8  RndMeth=Simplest
  Data Type Conversion4 : DataTypeConversion  OutDataTypeStr=uint16  RndMeth=Simplest
  Data Type Conversion5 : DataTypeConversion  OutDataTypeStr=int32  RndMeth=Simplest
  "EtherCAT Rx Var " : xpcethercatlib/EtherCAT PDO Receive  Priority=2  sig_name=Box 6 (ATRIAS 2.1 Hip (Medulla 1.5)).Measured Current.Amp Measured Current  sig_offset=2480  sig_type=int16  type_size=16  sig_dim=1  device_id=0  sample_time=0.000500
  EtherCAT Rx Var 1 : xpcethercatlib/EtherCAT PDO Receive  Priority=2  sig_name=Box 6 (ATRIAS 2.1 Hip (Medulla 1.5)).Power.Motor Voltage  sig_offset=2400  sig_type=uint16  type_size=16  sig_dim=1  device_id=0  sample_time=0.000500
  EtherCAT Rx Var 12 : xpcethercatlib/EtherCAT PDO Receive  Priority=2  sig_name=Box 6 (ATRIAS 2.1 Hip (Medulla 1.5)).Thermistors.Thermistor 0  sig_offset=2432  sig_type=uint16  type_size=16  sig_dim=1  device_id=0  sample_time=0.000500
  EtherCAT Rx Var 13 : xpcethercatlib/EtherCAT PDO Receive  Priority=2  sig_name=Box 6 (ATRIAS 2.1 Hip (Medulla 1.5)).Thermistors.Thermistor 1  sig_offset=2448  sig_type=uint16  type_size=16  sig_dim=1  device_id=0  sample_time=0.000500
  EtherCAT Rx Var 14 : xpcethercatlib/EtherCAT PDO Receive  Priority=2  sig_name=Box 6 (ATRIAS 2.1 Hip (Medulla 1.5)).Thermistors.Thermistor 2  sig_offset=2464  sig_type=uint16  type_size=16  sig_dim=1  device_id=0  sample_time=0.000500
  EtherCAT Rx Var 15 : xpcethercatlib/EtherCAT PDO Receive  Priority=2  sig_name=Box 6 (ATRIAS 2.1 Hip (Medulla 1.5)).uController Status.Counter  sig_offset=2328  sig_type=uint8  type_size=8  sig_dim=1  device_id=0  sample_time=0.000500
  EtherCAT Rx Var 16 : xpcethercatlib/EtherCAT PDO Receive  Priority=2  sig_name=Box 6 (ATRIAS 2.1 Hip (Medulla 1.5)).uController Status.Error Flags  sig_offset=2336  sig_type=uint8  type_size=8  sig_dim=1  device_id=0  sample_time=0.000500
  EtherCAT Rx Var 17 : xpcethercatlib/EtherCAT PDO Receive  Priority=2  sig_name=Box 6 (ATRIAS 2.1 Hip (Medulla 1.5)).uController Status.ID  sig_offset=2312  sig_type=uint8  type_size=8  sig_dim=1  device_id=0  sample_time=0.000500
  EtherCAT Rx Var 18 : xpcethercatlib/EtherCAT PDO Receive  Priority=2  sig_name=Box 6 (ATRIAS 2.1 Hip (Medulla 1.5)).uController Status.Limit Switch  sig_offset=2344  sig_type=uint8  type_size=8  sig_dim=1  device_id=0  sample_time=0.000500
  EtherCAT Rx Var 19 : xpcethercatlib/EtherCAT PDO Receive  Priority=2  sig_name=Box 6 (ATRIAS 2.1 Hip (Medulla 1.5)).uController Status.State  sig_offset=2320  sig_type=uint8  type_size=8  sig_dim=1  device_id=0  sample_time=0.000500
  EtherCAT Rx Var 2 : xpcethercatlib/EtherCAT PDO Receive  Priority=2  sig_name=Box 6 (ATRIAS 2.1 Hip (Medulla 1.5)).Incremental Encoder.Incremental Encoder  sig_offset=2496  sig_type=uint16  type_size=16  sig_dim=1  device_id=0  sample_time=0.000500
  EtherCAT Rx Var 3 : xpcethercatlib/EtherCAT PDO Receive  Priority=2  sig_name=Box 6 (ATRIAS 2.1 Hip (Medulla 1.5)).Hip Encoder.Timestamp  sig_offset=2384  sig_type=uint16  type_size=16  sig_dim=1  device_id=0  sample_time=0.000500
  EtherCAT Rx Var 4 : xpcethercatlib/EtherCAT PDO Receive  Priority=2  sig_name=Box 6 (ATRIAS 2.1 Hip (Medulla 1.5)).Hip Encoder.Encoder  sig_offset=2352  sig_type=uint32  type_size=32  sig_dim=1  device_id=0  sample_time=0.000500
  EtherCAT Rx Var 5 : xpcethercatlib/EtherCAT PDO Receive  Priority=2  sig_name=Box 6 (ATRIAS 2.1 Hip (Medulla 1.5)).Incremental Encoder.Incremental Encoder Timestamp  sig_offset=2512  sig_type=uint16  type_size=16  sig_dim=1  device_id=0  sample_time=0.000500
  EtherCAT Rx Var 6 : xpcethercatlib/EtherCAT PDO Receive  Priority=2  sig_name=Box 6 (ATRIAS 2.1 Hip (Medulla 1.5)).Power.Logic Voltage  sig_offset=2416  sig_type=uint16  type_size=16  sig_dim=1  device_id=0  sample_time=0.000500
  EtherCAT Tx Var 3 : xpcethercatlib/EtherCAT PDO Transmit   Priority=3  sig_name=Box 6 (ATRIAS 2.1 Hip (Medulla 1.5)).uControllerInput.Command  sig_offset=2312  sig_type=uint8  type_size=8  sig_dim=1  device_id=0  sample_time=0.000500
  EtherCAT Tx Var 4 : xpcethercatlib/EtherCAT PDO Transmit   Priority=3  sig_name=Box 6 (ATRIAS 2.1 Hip (Medulla 1.5)).uControllerInput.Counter  sig_offset=2320  sig_type=uint16  type_size=16  sig_dim=1  device_id=0  sample_time=0.000500
  EtherCAT Tx Var 5 : xpcethercatlib/EtherCAT PDO Transmit   Priority=3  sig_name=Box 6 (ATRIAS 2.1 Hip (Medulla 1.5)).uControllerInput.Motor Current  sig_offset=2336  sig_type=int32  type_size=32  sig_dim=1  device_id=0  sample_time=0.000500
  Mux5 : Mux  Inputs=3
  HipEncoder : Outport
  IncEncoder : Outport  Port=2
  LimitSwitch : Outport  Port=3
  ID : Outport  Port=4
  State : Outport  Port=5
  Counter : Outport  Port=6
  ErrorFlags : Outport  Port=7
  HipEncoderTimestamp : Outport  Port=8
  IncEncoderTimestamp : Outport  Port=9
  MotorVoltage : Outport  Port=10
  LogicVoltage : Outport  Port=11
  Thermistors : Outport  Port=12
  AmpMeasuredCurrent : Outport  Port=13
  wires:
  Data Type Conversion3/1 -> EtherCAT Tx Var 3/1
  Data Type Conversion4/1 -> EtherCAT Tx Var 4/1
  Data Type Conversion5/1 -> EtherCAT Tx Var 5/1
  MedullaCmd/1 -> Data Type Conversion3/1
  MedullaCounter/1 -> Data Type Conversion4/1
  MotorCmd/1 -> Data Type Conversion5/1
  EtherCAT Rx Var 5/1 -> IncEncoderTimestamp/1
  EtherCAT Rx Var 4/1 -> HipEncoder/1
  EtherCAT Rx Var 3/1 -> HipEncoderTimestamp/1
  EtherCAT Rx Var 2/1 -> IncEncoder/1
  EtherCAT Rx Var 15/1 -> Counter/1
  EtherCAT Rx Var 17/1 -> ID/1
  EtherCAT Rx Var 18/1 -> LimitSwitch/1
  EtherCAT Rx Var 19/1 -> State/1
  EtherCAT Rx Var 16/1 -> ErrorFlags/1
  EtherCAT Rx Var 6/1 -> LogicVoltage/1
  EtherCAT Rx Var 1/1 -> MotorVoltage/1
  EtherCAT Rx Var 12/1 -> Mux5/1
  EtherCAT Rx Var 13/1 -> Mux5/2
  EtherCAT Rx Var 14/1 -> Mux5/3
  "EtherCAT Rx Var "/1 -> AmpMeasuredCurrent/1
  Mux5/1 -> Thermistors/1

== system DAQ_lib_HallPositionTorque/DAQ Safety Stops IMU Elmo Amplifiers Position and Torque Control with Hall Sensors/DAQ/EtherCATNetwork/EtherCATRobotMicrostrain/HipMedulla_3R ==
  MedullaCmd : Inport
  MedullaCounter : Inport  Port=2
  MotorCmd : Inport  Port=3
  Data Type Conversion3 : DataTypeConversion  OutDataTypeStr=uint8  RndMeth=Simplest
  Data Type Conversion4 : DataTypeConversion  OutDataTypeStr=uint16  RndMeth=Simplest
  Data Type Conversion5 : DataTypeConversion  OutDataTypeStr=int32  RndMeth=Simplest
  "EtherCAT Rx Var " : xpcethercatlib/EtherCAT PDO Receive  Priority=2  sig_name=Box 5 (ATRIAS 2.1 Hip (Medulla 1.5)).Measured Current.Amp Measured Current  sig_offset=2264  sig_type=int16  type_size=16  sig_dim=1  device_id=0  sample_time=0.000500
  EtherCAT Rx Var 1 : xpcethercatlib/EtherCAT PDO Receive  Priority=2  sig_name=Box 5 (ATRIAS 2.1 Hip (Medulla 1.5)).Power.Motor Voltage  sig_offset=2184  sig_type=uint16  type_size=16  sig_dim=1  device_id=0  sample_time=0.000500
  EtherCAT Rx Var 12 : xpcethercatlib/EtherCAT PDO Receive  Priority=2  sig_name=Box 5 (ATRIAS 2.1 Hip (Medulla 1.5)).Thermistors.Thermistor 0  sig_offset=2216  sig_type=uint16  type_size=16  sig_dim=1  device_id=0  sample_time=0.000500
  EtherCAT Rx Var 13 : xpcethercatlib/EtherCAT PDO Receive  Priority=2  sig_name=Box 5 (ATRIAS 2.1 Hip (Medulla 1.5)).Thermistors.Thermistor 1  sig_offset=2232  sig_type=uint16  type_size=16  sig_dim=1  device_id=0  sample_time=0.000500
  EtherCAT Rx Var 14 : xpcethercatlib/EtherCAT PDO Receive  Priority=2  sig_name=Box 5 (ATRIAS 2.1 Hip (Medulla 1.5)).Thermistors.Thermistor 2  sig_offset=2248  sig_type=uint16  type_size=16  sig_dim=1  device_id=0  sample_time=0.000500
  EtherCAT Rx Var 15 : xpcethercatlib/EtherCAT PDO Receive  Priority=2  sig_name=Box 5 (ATRIAS 2.1 Hip (Medulla 1.5)).uController Status.Counter  sig_offset=2112  sig_type=uint8  type_size=8  sig_dim=1  device_id=0  sample_time=0.000500
  EtherCAT Rx Var 16 : xpcethercatlib/EtherCAT PDO Receive  Priority=2  sig_name=Box 5 (ATRIAS 2.1 Hip (Medulla 1.5)).uController Status.Error Flags  sig_offset=2120  sig_type=uint8  type_size=8  sig_dim=1  device_id=0  sample_time=0.000500
  EtherCAT Rx Var 17 : xpcethercatlib/EtherCAT PDO Receive  Priority=2  sig_name=Box 5 (ATRIAS 2.1 Hip (Medulla 1.5)).uController Status.ID  sig_offset=2096  sig_type=uint8  type_size=8  sig_dim=1  device_id=0  sample_time=0.000500
  EtherCAT Rx Var 18 : xpcethercatlib/EtherCAT PDO Receive  Priority=2  sig_name=Box 5 (ATRIAS 2.1 Hip (Medulla 1.5)).uController Status.Limit Switch  sig_offset=2128  sig_type=uint8  type_size=8  sig_dim=1  device_id=0  sample_time=0.000500
  EtherCAT Rx Var 19 : xpcethercatlib/EtherCAT PDO Receive  Priority=2  sig_name=Box 5 (ATRIAS 2.1 Hip (Medulla 1.5)).uController Status.State  sig_offset=2104  sig_type=uint8  type_size=8  sig_dim=1  device_id=0  sample_time=0.000500
  EtherCAT Rx Var 2 : xpcethercatlib/EtherCAT PDO Receive  Priority=2  sig_name=Box 5 (ATRIAS 2.1 Hip (Medulla 1.5)).Incremental Encoder.Incremental Encoder  sig_offset=2280  sig_type=uint16  type_size=16  sig_dim=1  device_id=0  sample_time=0.000500
  EtherCAT Rx Var 3 : xpcethercatlib/EtherCAT PDO Receive  Priority=2  sig_name=Box 5 (ATRIAS 2.1 Hip (Medulla 1.5)).Hip Encoder.Timestamp  sig_offset=2168  sig_type=uint16  type_size=16  sig_dim=1  device_id=0  sample_time=0.000500
  EtherCAT Rx Var 4 : xpcethercatlib/EtherCAT PDO Receive  Priority=2  sig_name=Box 5 (ATRIAS 2.1 Hip (Medulla 1.5)).Hip Encoder.Encoder  sig_offset=2136  sig_type=uint32  type_size=32  sig_dim=1  device_id=0  sample_time=0.000500
  EtherCAT Rx Var 5 : xpcethercatlib/EtherCAT PDO Receive  Priority=2  sig_name=Box 5 (ATRIAS 2.1 Hip (Medulla 1.5)).Incremental Encoder.Incremental Encoder Timestamp  sig_offset=2296  sig_type=uint16  type_size=16  sig_dim=1  device_id=0  sample_time=0.000500
  EtherCAT Rx Var 6 : xpcethercatlib/EtherCAT PDO Receive  Priority=2  sig_name=Box 5 (ATRIAS 2.1 Hip (Medulla 1.5)).Power.Logic Voltage  sig_offset=2200  sig_type=uint16  type_size=16  sig_dim=1  device_id=0  sample_time=0.000500
  EtherCAT Tx Var 3 : xpcethercatlib/EtherCAT PDO Transmit   Priority=3  sig_name=Box 5 (ATRIAS 2.1 Hip (Medulla 1.5)).uControllerInput.Command  sig_offset=2096  sig_type=uint8  type_size=8  sig_dim=1  device_id=0  sample_time=0.000500
  EtherCAT Tx Var 4 : xpcethercatlib/EtherCAT PDO Transmit   Priority=3  sig_name=Box 5 (ATRIAS 2.1 Hip (Medulla 1.5)).uControllerInput.Counter  sig_offset=2104  sig_type=uint16  type_size=16  sig_dim=1  device_id=0  sample_time=0.000500
  EtherCAT Tx Var 5 : xpcethercatlib/EtherCAT PDO Transmit   Priority=3  sig_name=Box 5 (ATRIAS 2.1 Hip (Medulla 1.5)).uControllerInput.Motor Current  sig_offset=2120  sig_type=int32  type_size=32  sig_dim=1  device_id=0  sample_time=0.000500
  Mux5 : Mux  Inputs=3
  HipEncoder : Outport
  IncEncoder : Outport  Port=2
  LimitSwitch : Outport  Port=3
  ID : Outport  Port=4
  State : Outport  Port=5
  Counter : Outport  Port=6
  ErrorFlags : Outport  Port=7
  HipEncoderTimestamp : Outport  Port=8
  IncEncoderTimestamp : Outport  Port=9
  MotorVoltage : Outport  Port=10
  LogicVoltage : Outport  Port=11
  Thermistors : Outport  Port=12
  AmpMeasuredCurrent : Outport  Port=13
  wires:
  Data Type Conversion3/1 -> EtherCAT Tx Var 3/1
  Data Type Conversion4/1 -> EtherCAT Tx Var 4/1
  Data Type Conversion5/1 -> EtherCAT Tx Var 5/1
  MedullaCmd/1 -> Data Type Conversion3/1
  MedullaCounter/1 -> Data Type Conversion4/1
  MotorCmd/1 -> Data Type Conversion5/1
  EtherCAT Rx Var 5/1 -> IncEncoderTimestamp/1
  EtherCAT Rx Var 4/1 -> HipEncoder/1
  EtherCAT Rx Var 3/1 -> HipEncoderTimestamp/1
  EtherCAT Rx Var 2/1 -> IncEncoder/1
  EtherCAT Rx Var 15/1 -> Counter/1
  EtherCAT Rx Var 17/1 -> ID/1
  EtherCAT Rx Var 18/1 -> LimitSwitch/1
  EtherCAT Rx Var 19/1 -> State/1
  EtherCAT Rx Var 16/1 -> ErrorFlags/1
  EtherCAT Rx Var 6/1 -> LogicVoltage/1
  EtherCAT Rx Var 1/1 -> MotorVoltage/1
  EtherCAT Rx Var 12/1 -> Mux5/1
  EtherCAT Rx Var 13/1 -> Mux5/2
  EtherCAT Rx Var 14/1 -> Mux5/3
  "EtherCAT Rx Var "/1 -> AmpMeasuredCurrent/1
  Mux5/1 -> Thermistors/1
